simulink model "twolink_simulink_analysis"  (R2015a)
settings: Solver=ode45  StartTime=solversettings.t_start  StopTime=solversettings.t_stop  MaxStep=solversettings.t_sample  RelTol=solversettings.rel_tol  AbsTol=solversettings.abs_tol
values from neighbouring files (symbols this model uses):
  solversettings =     [settings.mat]
libraries: robotlib x5, simulink x2
settings Model: Creator=jwcjdenissen  LastModifiedBy=jwcjdenissen
settings DataIOCC: LimitDataPoints=off  SaveOutput=off  SaveTime=off
settings DebuggingCC: UnconnectedInputMsg=none  UnconnectedOutputMsg=none  UnconnectedLineMsg=none

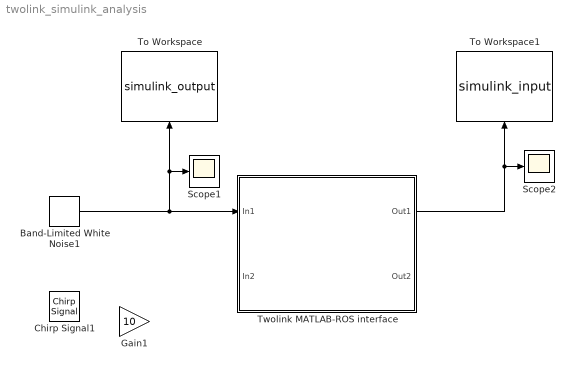
== system twolink_simulink_analysis ==
  Band-Limited White Noise1 : simulink/Sources/Band-Limited White Noise  Cov=[0.01]  Ts=solversettings.t_sample  seed=[round(rand*10000)]
  Chirp Signal1 : simulink/Sources/Chirp Signal  f1=0.01  T=10  f2=100
  Gain1 : Gain  Gain=10
  Scope1 : Scope
      settings: TimeRange=1.600000000000001  YMin=-22.5  YMax=25
  Scope2 : Scope
      settings: TimeRange=2  YMin=-0.725  YMax=-0.525  SaveName=ScopeData2
  To Workspace : ToWorkspace  SaveFormat=Timeseries  SampleTime=-1
  To Workspace1 : ToWorkspace  VariableName=simulink_input  SaveFormat=Timeseries  SampleTime=-1
  Twolink MATLAB-ROS interface : Subsystem
  wires:
  Band-Limited White Noise1/1 -> Scope1/1, To Workspace/1, Twolink MATLAB-ROS interface/1(In1)
  Twolink MATLAB-ROS interface/1(Out1) -> Scope2/1, To Workspace1/1

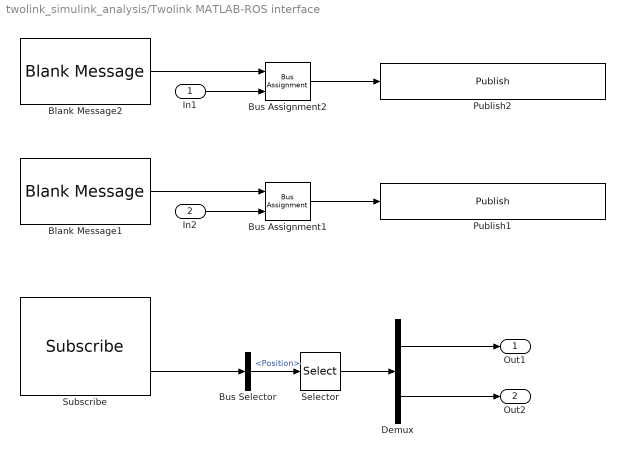
== system twolink_simulink_analysis/Twolink MATLAB-ROS interface ==
  In1 : Inport
  In2 : Inport  Port=2
  Blank Message1 : robotlib/Blank Message  SourceLibraryInfo=This block requires Robotics System Toolbox  messageType=std_msgs/Float64  SampleTime=inf
  Blank Message2 : robotlib/Blank Message  SourceLibraryInfo=This block requires Robotics System Toolbox  messageType=std_msgs/Float64  SampleTime=inf
  Bus Assignment1 : BusAssignment  AssignedSignals=Data
  Bus Assignment2 : BusAssignment  AssignedSignals=Data
  Bus Selector : BusSelector  OutputSignals=Position
  Demux : Demux  Outputs=2
  Publish1 : robotlib/Publish  SourceLibraryInfo=This block requires Robotics System Toolbox  topicSource=Specify your own  topic=/twolink/joint_2_effort_controller/command  messageType=std_msgs/Float64  messageQueueLength=1
  Publish2 : robotlib/Publish  SourceLibraryInfo=This block requires Robotics System Toolbox  topicSource=Specify your own  topic=/twolink/joint_1_effort_controller/command  messageType=std_msgs/Float64  messageQueueLength=1
  Selector : Selector  InputPortWidth=128  Indices=[1 2]
  Subscribe : robotlib/Subscribe  SourceLibraryInfo=This block requires Robotics System Toolbox  topicSource=Specify your own  topic=/twolink/joint_states  messageType=sensor_msgs/JointState  sampleTime=-1  messageQueueLength=1
  Out1 : Outport
  Out2 : Outport  Port=2
  wires:
  Blank Message1/1 -> Bus Assignment1/1
  Bus Assignment1/1 -> Publish1/1
  Blank Message2/1 -> Bus Assignment2/1
  Bus Assignment2/1 -> Publish2/1
  In1/1 -> Bus Assignment2/2
  In2/1 -> Bus Assignment1/2
  Subscribe/2 -> Bus Selector/1
  Bus Selector/1 -> Selector/1  "<Position>"
  Selector/1 -> Demux/1
  Demux/1 -> Out1/1
  Demux/2 -> Out2/1
